simulink model "wireless"  (R2016a)
settings: Solver=ode45  StartTime=0.0  StopTime=2  RelTol=1e-3
InitFcn:
  | clear functions
undefined symbols (not defined in the file or in its folder): WLAN
libraries: truetime x3
settings Model: ExtModeAutoUpdateStatusClock=off  Creator=anton  LastModifiedBy=ZEYU
settings DataIOCC: LimitDataPoints=on  SaveFormat=Array  SaveOutput=off  SaveTime=off
settings OptimizationCC: BlockReduction=off  BooleanDataType=off  ExpressionDepthLimit=2147483647
settings DebuggingCC: SaveWithParameterizedLinksMsg=none  UnderspecifiedInitializationDetection=Classic  MergeDetectMultiDrivingBlocksExec=none  SignalResolutionControl=TryResolveAllWithWarning  MultiTaskDSMMsg=warning  MultiTaskCondExecSysMsg=none  FcnCallInpInsideContextMsg=EnableAllAsWarning  StateNameClashWarn=warning
settings HardwareCC: ProdBitPerPointer=32  ProdLargestAtomicFloat=None  ProdIntDivRoundTo=Undefined  ProdEndianess=Unspecified  ProdWordSize=32  ProdHWDeviceType=32-bit Generic  TargetUnknown=on
settings ModelReferenceCC: PropagateSignalLabelsOutOfModel=off
settings GRTTargetCC: TargetFcnLib=ansi_tfl_tmw.mat  CombineOutputUpdateFcns=off  GRTInterface=on

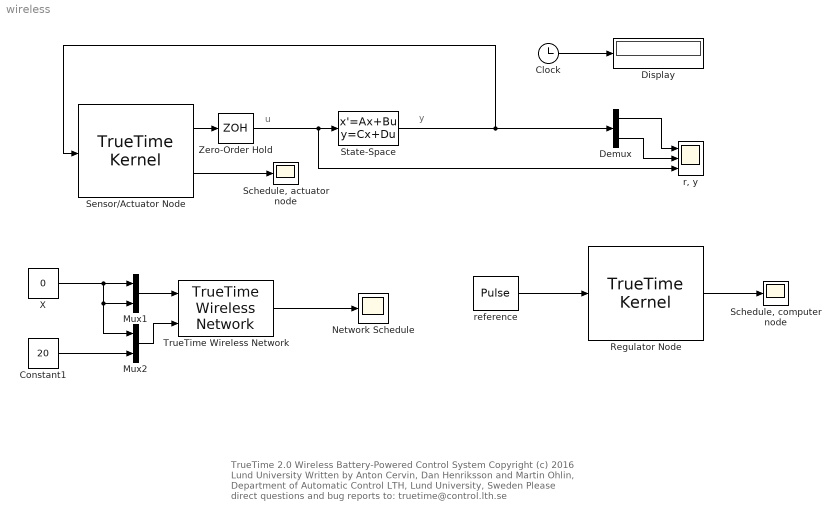
== system wireless ==
  note: u
  note: y
  note: TrueTime 2.0  Wireless Battery-Powered Control System
      | Copyright (c) 2016 Lund University
      | Written by Anton Cervin, Dan Henriksson and Martin Ohlin,
      | Department of Automatic Control LTH, Lund University, Sweden
      | Please direct questions and bug reports to: truetime@control.lth.se
  Clock : Clock
  Constant1 : Constant  Value=20
  Demux : Demux  Outputs=2
  Display : Display
  Mux1 : Mux  Inputs=2
  Mux2 : Mux  Inputs=2
  Network Schedule : Scope
  Regulator Node : truetime/TrueTime Kernel  sfun=regulator_init  args=[]  ninputsoutputs=[1 0]  ntriggers=0  trigtype=falling  nwnodenbr=2  clockoffsetdrift=[0 0]  schedoutput=on  battery=off  poweroutput=off  label=1: 2
  "Schedule, actuator node" : Scope
  "Schedule, computer node" : Scope
  Sensor/Actuator Node : truetime/TrueTime Kernel  sfun=actuator_init  args=[]  ninputsoutputs=[2 1]  ntriggers=0  trigtype=falling  nwnodenbr=1  clockoffsetdrift=[0 0]  schedoutput=on  battery=off  poweroutput=off  label=1: 1
  State-Space : StateSpace  A=[0 1; 0 -1]  B=[0 1000]'  C=[1 0; 0 1]  D=[0 0]'  X0=[1 1]'
  TrueTime Wireless Network : truetime/TrueTime Wireless  Network  nwtype=802.11b (WLAN)  nwnbr=1  nnodes=2  rate=800000  minsize=272  transpower=30  threshold=-48  use_pathloss_function=default  pathloss=3.5  acktimeout=0.00004  retrylimit=5  error_threshold=0.03  lossprob=0.3  seed=0  scheduleoutput=on  poweroutput=off
  X : Constant  Value=0
  Zero-Order Hold : ZeroOrderHold  SampleTime=0.01
  "r, y" : Scope  NumInputPorts=3
  reference : DiscretePulseGenerator  PulseType=Time based  Period=1.2  PulseWidth=50
  wires:
  Clock/1 -> Display/1
  X/1 -> Mux1/1, Mux1/2, Mux2/1
  Constant1/1 -> Mux2/2
  Mux1/1 -> TrueTime Wireless Network/1
  Mux2/1 -> TrueTime Wireless Network/2
  TrueTime Wireless Network/1 -> Network Schedule/1
  Sensor/Actuator Node/2 -> "Schedule, actuator node"/1
  Regulator Node/1 -> "Schedule, computer node"/1
  reference/1 -> Regulator Node/1
  State-Space/1 -> Sensor/Actuator Node/1, Demux/1
  Sensor/Actuator Node/1 -> Zero-Order Hold/1
  Demux/2 -> "r, y"/2
  Demux/1 -> "r, y"/1
  Zero-Order Hold/1 -> State-Space/1, "r, y"/3
